simulink subsystem "ZAxisSubsystem"  (R2023b)
settings: Solver=VariableStepAuto  StartTime=0.0  StopTime=10.0  RelTol=1e-3
values from neighbouring files (symbols this model uses):
  Az = 0.0    (= 0)    [drone_input_params.m]
  g = 9.81    [drone_input_params.m]
  m = weight/g    (= 0.815494393476)    [drone_input_params.m]
settings Model: Creator=FRESH  LastModifiedBy=FRESH

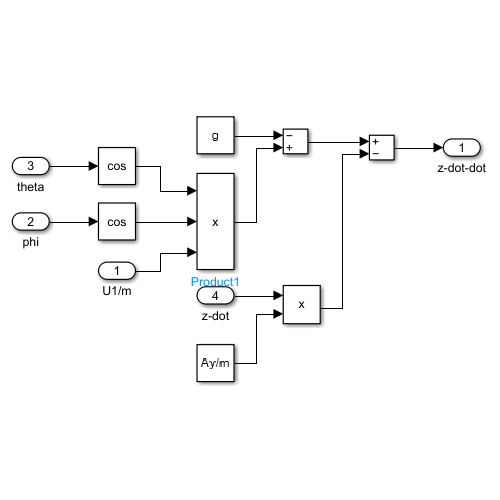
[thumbnail: Simulink's stored preview of the top-level diagram]
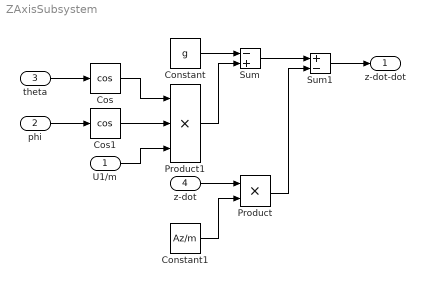
== system ZAxisSubsystem ==
  U1/m : Inport
  phi : Inport  Port=2
  theta : Inport  Port=3
  z-dot : Inport  Port=4
  Constant : Constant  Value=g
  Constant1 : Constant  Value=Az/m
  Cos : Trigonometry  Operator=cos
  Cos1 : Trigonometry  Operator=cos
  Product : Product
  Product1 : Product  Inputs=3
  Sum : Sum  Inputs=-+
  Sum1 : Sum  Inputs=+-
  z-dot-dot : Outport
  wires:
  Cos1/1 -> Product1/2
  theta/1 -> Cos/1
  Product/1 -> Sum1/2
  phi/1 -> Cos1/1
  Constant/1 -> Sum/1
  U1/m/1 -> Product1/3
  Cos/1 -> Product1/1
  Product1/1 -> Sum/2
  z-dot/1 -> Product/1
  Constant1/1 -> Product/2
  Sum/1 -> Sum1/1
  Sum1/1 -> z-dot-dot/1
